simulink model "cube2"  (R2014b)
settings: Solver=ode45  StartTime=0.0  StopTime=4  MaxStep=0.01  RelTol=1e-3
values from neighbouring files (symbols this model uses):
  A = [a11, a12, a13; a21, a22, a23; a31, a32, a33]    [gs.m]
  B = [b1; b2; b3]    [gs.m]
  C = [1 0 0; 0 1 0; 0 0 1]    [gs.m]
  D = [0; 0; 0]    [gs.m]
  eta = 0.9    [gs.m]
  g = 9.82    [gs.m]
  Ik = 0.015    [gs.m]
  Is = Ms*rs^2/2    (= 0.0005625)    [gs.m]
  J = 138E-7    (= 1.38e-05)    [gs.m]
  K_emf = 1/158    (= 0.00632911392405)    [gs.m]
  Kt = 60.3*10^-3    (= 0.0603)    [gs.m]
  L = 0.329E-3    (= 0.000329)    [gs.m]
  l = 0.17    [gs.m]
  max_current = 20    [gs.m]
  max_voltage = 48    [gs.m]
  Mtot = alu_mass + motor_mass + motor_power + arduino_mass + extra + M_s    (= 1.35)    [gs.m]
  Rm = 1.16    [gs.m]
  X0 = x0    [gs.m]
undefined symbols (not defined in the file or in its folder): etaGear, Gear, K, Ts
libraries: simulink x1
settings Model: Creator=MikaelSjostedt  LastModifiedBy=MikaelSjostedt
settings OptimizationCC: OptimizeModelRefInitCode=on  LifeSpan=1
settings DebuggingCC: UnderspecifiedInitializationDetection=Classic  MergeDetectMultiDrivingBlocksExec=none
settings HardwareCC: ProdBitPerInt=16  ProdBitPerPointer=8  ProdIntDivRoundTo=Zero  ProdEndianess=LittleEndian  ProdWordSize=8  ProdHWDeviceType=Atmel->AVR
settings RTWCC: SystemTargetFile=realtime.tlc  GenerateMakefile=off  TemplateMakefile=realtime.tmf  Description=Run on Target Hardware  RTWVerbose=off  ProcessScript=realtime_make_rtw_hook
settings CodeAppCC: IgnoreCustomStorageClasses=off
settings STFCustomTargetCC: TargetLibSuffix=.a  GenerateSampleERTMain=on  CombineOutputUpdateFcns=on  ERTCustomFileBanners=on  SupportContinuousTime=off  SupportNonInlinedSFcns=off  MATLABClassNameForMDSCustomization=Simulink.SoftwareTarget.ERTCustomization  GRTInterface=off  SystemTargetFile=realtime.tlc
settings ERTTargetCC: GenerateSampleERTMain=on  ParMdlRefBuildCompliant=off  CompOptLevelCompliant=off  ConcurrentExecutionCompliant=off  ERTFirstTimeCompliant=off  ModelStepFunctionPrototypeControlCompliant=off  CPPClassGenCompliant=off  InlinedParameterPlacement=NonHierarchical  ERTCustomFileTemplate=realtime_file_process.tlc

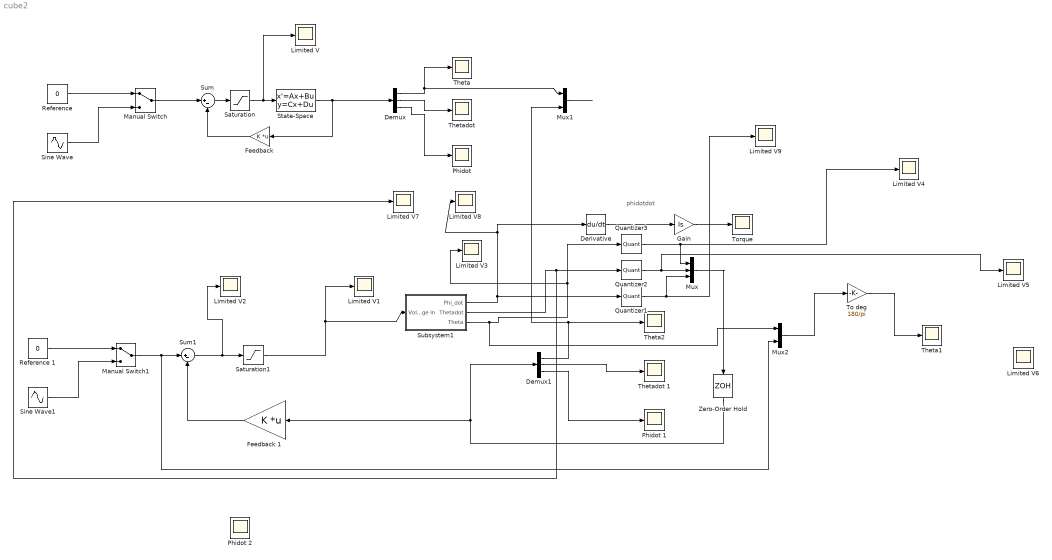
== system cube2 ==
  note: phidotdot
  Demux : Demux  Outputs=3
  Demux1 : Demux  Outputs=3
  Derivative : Derivative
  "Feedback " : Gain  Gain=K  Multiplication=Matrix(K*u)
  Feedback 1 : Gain  Gain=K  Multiplication=Matrix(K*u)
  Gain : Gain  Gain=Is
  Limited V{,1..9} (10 alike) : Scope
      Limited V settings: SaveName=ScopeVoltage
      Limited V1 settings: SaveName=ScopeVoltage1
      Limited V2 settings: SaveName=ScopeVoltage2
      Limited V3 settings: SaveName=ScopeVoltage3
      Limited V4 settings: SaveName=ScopeVoltage4
      Limited V5 settings: SaveName=ScopeVoltage5
      Limited V6 settings: SaveName=ScopeVoltage6
      Limited V7 settings: SaveName=ScopeVoltage7
      Limited V8 settings: SaveName=ScopeVoltage8
      Limited V9 settings: SaveName=ScopeVoltage9
  Manual Switch : ManualSwitch
  Manual Switch1 : ManualSwitch
  Mux : Mux  Inputs=3
  Mux1 : Mux  Inputs=2
  Mux2 : Mux  Inputs=2
  "Phidot " : Scope
      settings: SaveName=ScopeData3
  Phidot 1 : Scope
      settings: SaveName=ScopeData2
  Phidot 2 : Scope
      settings: SaveName=ScopeData5
  Quantizer1 : Quantizer  QuantizationInterval=1/(1024/(2*pi))
  Quantizer2 : Quantizer  QuantizationInterval=1/(2^16/(2*pi))
  Quantizer3 : Quantizer  QuantizationInterval=1/(2^16/(2*pi))
  "Reference " : Constant  Value=0
  Reference 1 : Constant  Value=0
  Saturation : Saturate  UpperLimit=48  LowerLimit=-48
  Saturation1 : Saturate  UpperLimit=max_voltage  LowerLimit=-max_voltage
  Sine Wave : Sin  SampleTime=0
  Sine Wave1 : Sin  Amplitude=0.2618  SampleTime=0
  State-Space : StateSpace  A=A  B=B  C=C  D=D  X0=X0
  Subsystem1 : Subsystem
  Sum : Sum  Inputs=|+-
  Sum1 : Sum  Inputs=|+-
  Theta : Scope
      settings: SaveName=ScopeTheta
  Theta1 : Scope
      settings: SaveName=ScopeTheta2
  Theta2 : Scope
      settings: SaveName=ScopeTheta1
  "Thetadot " : Scope
  Thetadot 1 : Scope
      settings: SaveName=ScopeData4
  "To deg " : Gain  Gain=180/pi
  Torque : Scope
      settings: SaveName=ScopeData6
  Zero-Order Hold : ZeroOrderHold  SampleTime=Ts
  wires:
  Demux/2 -> "Thetadot "/1
  Demux/1 -> Theta/1, Mux1/1
  Demux/3 -> "Phidot "/1
  State-Space/1 -> "Feedback "/1, Demux/1
  "Feedback "/1 -> Sum/2
  Sum/1 -> Saturation/1
  Saturation/1 -> Limited V/1, State-Space/1
  Manual Switch1/1 -> Mux2/2, Sum1/1
  Demux1/2 -> Thetadot 1/1
  Demux1/1 -> Theta2/1, Mux1/2
  Demux1/3 -> Phidot 1/1
  Feedback 1/1 -> Sum1/2
  Sum1/1 -> Limited V2/1, Saturation1/1
  Saturation1/1 -> Limited V1/1, Subsystem1/1("Voltage in ")
  Subsystem1/3(Theta) -> Mux2/1, Quantizer3/1, Limited V3/1
  Subsystem1/2("Thetadot ") -> Limited V7/1, Quantizer2/1
  Subsystem1/1(Phi_dot) -> Derivative/1, Limited V8/1, Quantizer1/1
  Mux1/1 -> ?
  Derivative/1 -> Gain/1
  Gain/1 -> Torque/1
  Manual Switch/1 -> Sum/1
  "Reference "/1 -> Manual Switch/1
  Sine Wave/1 -> Manual Switch/2
  Reference 1/1 -> Manual Switch1/1
  Sine Wave1/1 -> Manual Switch1/2
  Mux2/1 -> "To deg "/1
  "To deg "/1 -> Theta1/1
  Mux/1 -> Zero-Order Hold/1
  Quantizer1/1 -> Limited V9/1, Mux/3
  Quantizer2/1 -> Limited V5/1, Mux/2
  Quantizer3/1 -> Mux/1, Limited V4/1
  Zero-Order Hold/1 -> Feedback 1/1, Demux1/1

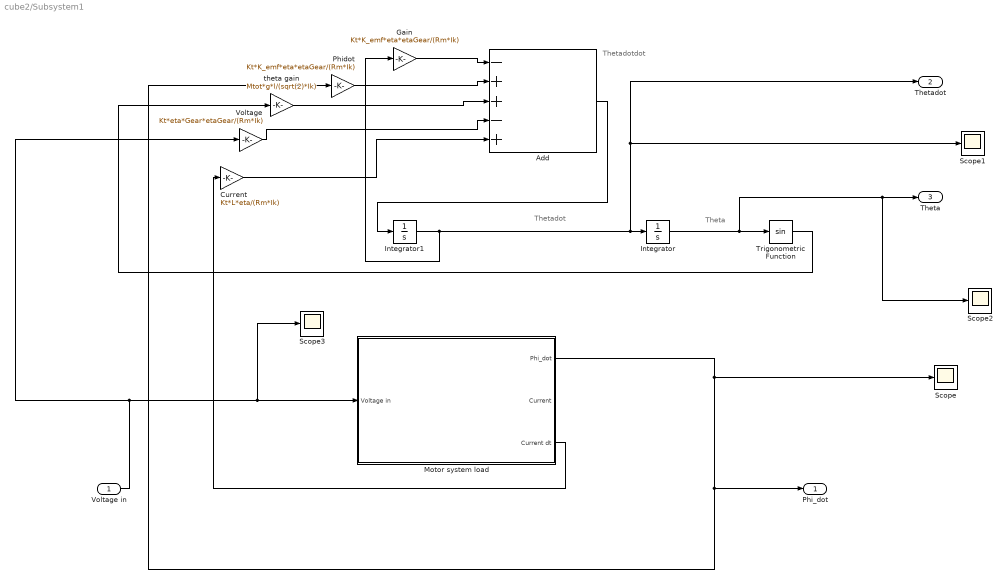
== system cube2/Subsystem1 ==
  note: Theta
  note: Thetadot
  note: Thetadotdot
  "Voltage in " : Inport
  Add : Sum  Inputs=-++-+
  Current : Gain  Gain=Kt*L*eta/(Rm*Ik)
  Gain : Gain  Gain=Kt*K_emf*eta*etaGear/(Rm*Ik)
  Integrator : Integrator  InitialCondition=X0(1)  LimitOutput=on  UpperSaturationLimit=pi/2  LowerSaturationLimit=-pi/2
  Integrator1 : Integrator
  "Motor system load " : Subsystem
  Phidot : Gain  Gain=Kt*K_emf*eta*etaGear/(Rm*Ik)
  Scope{,1..3} (4 alike) : Scope
      Scope settings: SaveName=ScopeData10
      Scope1 settings: SaveName=ScopeData11
      Scope2 settings: SaveName=ScopeData12
      Scope3 settings: SaveName=ScopeData13
  Trigonometric Function : Trigonometry
  Voltage : Gain  Gain=Kt*eta*Gear*etaGear/(Rm*Ik)
  theta gain : Gain  Gain=Mtot*g*l/(sqrt(2)*Ik)
  Phi_dot : Outport
  "Thetadot " : Outport  Port=2
  Theta : Outport  Port=3
  wires:
  Trigonometric Function/1 -> theta gain/1
  Integrator/1 -> Scope2/1, Theta/1, Trigonometric Function/1
  Integrator1/1 -> Gain/1, "Thetadot "/1, Scope1/1, Integrator/1
  Add/1 -> Integrator1/1
  Voltage/1 -> Add/4
  Phidot/1 -> Add/2
  theta gain/1 -> Add/3
  Gain/1 -> Add/1
  "Voltage in "/1 -> Voltage/1, Scope3/1, "Motor system load "/1("Voltage in ")
  "Motor system load "/3("Current dt ") -> Current/1
  Current/1 -> Add/5
  "Motor system load "/1(Phi_dot) -> Phi_dot/1, Phidot/1, Scope/1

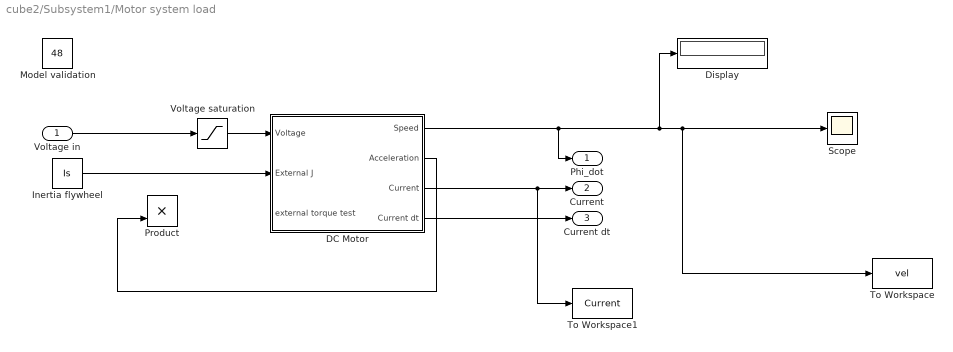
== system cube2/Subsystem1/Motor system load  ==
  "Voltage in " : Inport
  DC Motor : Subsystem
  Display : Display
  "Inertia flywheel " : Constant  Value=Is
  "Model validation " : Constant  Value=48
  Product : Product
  Scope : Scope
  To Workspace : ToWorkspace  VariableName=vel  SampleTime=-1
  To Workspace1 : ToWorkspace  VariableName=Current  SampleTime=-1
  Voltage saturation : Saturate  UpperLimit=max_voltage  LowerLimit=-max_voltage
  Phi_dot : Outport
  Current : Outport  Port=2
  "Current dt " : Outport  Port=3
  wires:
  DC Motor/1(" Speed") -> Phi_dot/1, Display/1, To Workspace/1, Scope/1
  Voltage saturation/1 -> DC Motor/1(Voltage)
  DC Motor/2(Acceleration) -> Product/2
  DC Motor/3(Current) -> To Workspace1/1, Current/1
  DC Motor/4(Current dt) -> "Current dt "/1
  "Voltage in "/1 -> Voltage saturation/1
  "Inertia flywheel "/1 -> DC Motor/2(External J)

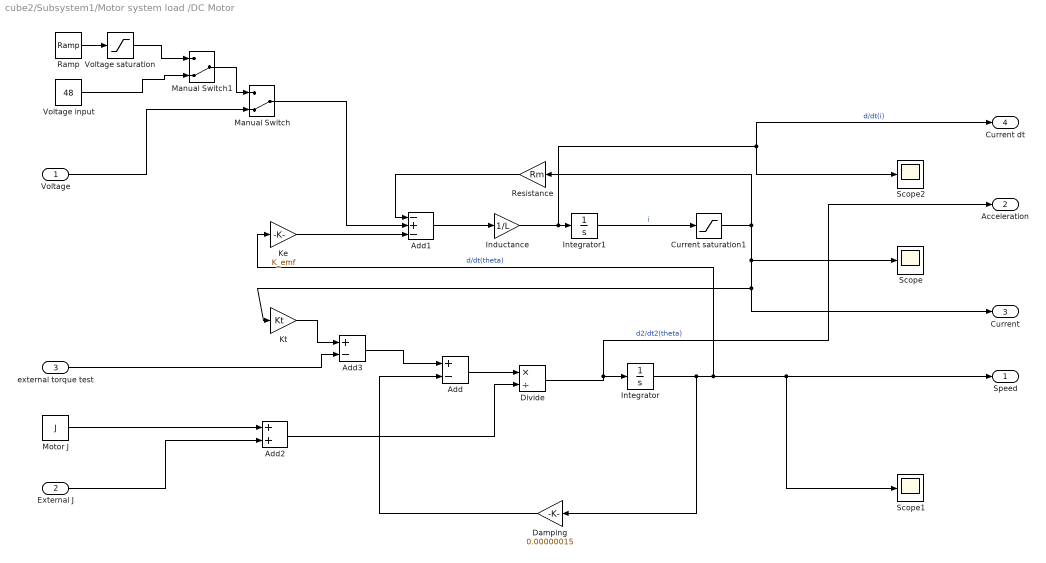
== system cube2/Subsystem1/Motor system load /DC Motor ==
  Voltage : Inport
  External J : Inport  Port=2
  "external torque test " : Inport  Port=3
  Add : Sum  Inputs=+-
  Add1 : Sum  Inputs=-+-
  Add2 : Sum
  Add3 : Sum  Inputs=+-
  Current saturation1 : Saturate  UpperLimit=max_current  LowerLimit=-max_current
  Damping : Gain  Gain=0.00000015
  Divide : Product  Inputs=*/
  Inductance : Gain  Gain=1/L
  Integrator : Integrator  InitialCondition=X0(2)
  Integrator1 : Integrator
  Ke : Gain  Gain=K_emf
  Kt : Gain  Gain=Kt
  Manual Switch : ManualSwitch  CurrentSetting=0
  Manual Switch1 : ManualSwitch  CurrentSetting=0
  "Motor J " : Constant  Value=J
  Ramp : simulink/Sources/Ramp  slope=100  start=0  X0=0
  Resistance : Gain  Gain=Rm
  Scope : Scope
      settings: SaveName=ScopeData7
  Scope1 : Scope
      settings: SaveName=ScopeData8
  Scope2 : Scope
      settings: SaveName=ScopeData9
  "Voltage input " : Constant  Value=48
  Voltage saturation : Saturate  UpperLimit=max_voltage  LowerLimit=-max_voltage
  " Speed" : Outport
  Acceleration : Outport  Port=2
  Current : Outport  Port=3
  Current dt : Outport  Port=4
  wires:
  Integrator1/1 -> Current saturation1/1  "i"
  Inductance/1 -> Integrator1/1, Scope2/1, Current dt/1  "d/dt(i)"
  Divide/1 -> Acceleration/1, Integrator/1  "d2/dt2(theta)"
  Integrator/1 -> Ke/1, Scope1/1, " Speed"/1, Damping/1  "d/dt(theta)"
  Add1/1 -> Inductance/1
  Add/1 -> Divide/1
  Damping/1 -> Add/2
  Kt/1 -> Add3/1
  Resistance/1 -> Add1/1
  Ke/1 -> Add1/3
  Add3/1 -> Add/1
  "external torque test "/1 -> Add3/2
  Current saturation1/1 -> Scope/1, Current/1, Kt/1, Resistance/1
  Ramp/1 -> Voltage saturation/1
  Voltage/1 -> Manual Switch/2
  "Voltage input "/1 -> Manual Switch1/2
  Manual Switch1/1 -> Manual Switch/1
  Voltage saturation/1 -> Manual Switch1/1
  Manual Switch/1 -> Add1/2
  "Motor J "/1 -> Add2/1
  External J/1 -> Add2/2
  Add2/1 -> Divide/2
